simulink model "Microgrid_PV_WG_Bat_EV_j_22b"  (R2022b)
settings: Solver=VariableStepAuto  StartTime=0.0  StopTime=1  RelTol=1e-3
undefined symbols (not defined in the file or in its folder): Acid, Ion, Lead, Lithium
libraries: slpidlib x35, spsabctodq0Lib x23, spsSeriesRLCBranchLib x19, spsCurrentMeasurementLib x13, spsVoltageMeasurementLib x11, spsThreePhaseVIMeasurementLib x10, spsPLL3phLib x9, spsThreePhaseSeriesRLCBranchLib x9, spsPower3phInstantaneousLib x8, spsIGBTDiodeLib x8, spsUniversalBridgeLib x7, spsPWMGeneratorDCDCLib x6
(part 4 of 5)

== system Microgrid_PV_WG_Bat_EV_j_22b/逆变器整流1/controller2 ==
  note: abc2dq
  Udc : Inport
  Udc_ref : Inport  Port=2
  Vabc : Inport  Port=3
  Iabc : Inport  Port=4
  Constant : Constant  Commented=on  Value=600
  Constant4 : Constant  Value=0
  Demux2 : Demux  Outputs=3
  Demux3 : Demux  Outputs=3
  Demux4 : Demux  Outputs=3
  Gain6 : Gain  Gain=2*pi*50*(7e-3)
  Gain7 : Gain  Gain=2*pi*50*(7e-3)
  Gain9 : Gain  Gain=0.0017
  Mux1 : Mux  Inputs=3
  PID 3 : slpidlib/PID Controller  Controller=PID  Form=Parallel  TimeDomain=Discrete-time  UseExternalTs=off  SampleTime=1e-5  IntegratorMethod=Forward Euler  FilterMethod=Forward Euler  ControllerParametersSource=internal  P=2  I=70  UseKiTs=off  D=0  N=100  UseFilter=on  TunerSelectOption=Transfer Function Based (PID Tuner App)  InitialConditionSource=internal  InitialConditionForIntegrator=0  InitialConditionForFilter=0  DifferentiatorICPrevScaledInput=0  ExternalReset=none  TrackingMode=off  Kt=1  LimitOutput=off  SatLimitsSource=internal  UpperSaturationLimit=inf  LowerSaturationLimit=-inf  LinearizeAsGain=on  AntiWindupMode=none  Kb=1  LimitIntegrator=off  UpperIntegratorSaturationLimit=inf  LowerIntegratorSaturationLimit=-inf  POutMin=[]  POutMax=[]  IOutMin=[]  IOutMax=[]  DOutMin=[]  DOutMax=[]  NOutMin=[]  NOutMax=[]  SumOutMin=[]  SumOutMax=[]  SaturationOutMin=[]  SaturationOutMax=[]  PParamMin=[]  PParamMax=[]  IParamMin=[]  IParamMax=[]  DParamMin=[]  DParamMax=[]  NParamMin=[]  NParamMax=[]  KbParamMin=[]  KbParamMax=[]  KtParamMin=[]  KtParamMax=[]  KbOutMin=[]  KbOutMax=[]  KtOutMin=[]  KtOutMax=[]  IntegratorOutMin=[]  IntegratorOutMax=[]  FilterOutMin=[]  FilterOutMax=[]  SumI1OutMin=[]  SumI1OutMax=[]  SumI2OutMin=[]  SumI2OutMax=[]  SumI3OutMin=[]  SumI3OutMax=[]  SumI4OutMin=[]  SumI4OutMax=[]  SumDOutMin=[]  SumDOutMax=[]  DifferentiatorOutMin=[]  DifferentiatorOutMax=[]  FilterDiffOutCoefMin=[]  FilterDiffOutCoefMax=[]  ReciprocalOutMin=[]  ReciprocalOutMax=[]  SumDenOutMin=[]  SumDenOutMax=[]  SumNumOutMin=[]  SumNumOutMax=[]  DivideOutMin=[]  DivideOutMax=[]  UdiffTsProdOutMin=[]  UdiffTsProdOutMax=[]  NTsProdOutMin=[]  NTsProdOutMax=[]  UintegralTsProdOutMin=[]  UintegralTsProdOutMax=[]  UngainTsProdOutMin=[]  UngainTsProdOutMax=[]  IntegratorContinuousStateAttributes=''  IntegratorStateMustResolveToSignalObject=off  IntegratorRTWStateStorageClass=Auto  FilterContinuousStateAttributes=''  FilterStateMustResolveToSignalObject=off  FilterRTWStateStorageClass=Auto  ParallelPVariant=InternalParameters  IdealPVariant=Disabled  IVariant=InternalParameters  DVariant=InternalParameters  IntegratorVariant=Discrete  SatVariant=Disabled  AWVariant=Passthrough  PCopyVariant=Disabled  TRVariant=Disabled  FdbkBlocksVariant=Forward  IdealPFdbkVariant=Disabled  SatFdbkVariant=Disabled  DerivativeFilterVariant=ForwardEulerFilter  NVariant=InternalParameters  NCopyVariant=Disabled  FilterICVariant=InternalICsFilter  IntegratorICVariant=InternalICs  ExternalResetVariant=Disabled  TRSumVariant=Passthrough  SumFdbkVariant=Disabled  SumVariant=Sum_PID  TsampFilterVariant=InternalTs  TsampNgainVariant=Passthrough  TsampIntegralVariant=Disabled_SignalSpec  ExternalSaturationOutDataTypeStr=Inherit: Same as second input
  PID 4 : slpidlib/PID Controller  Controller=PID  Form=Parallel  TimeDomain=Discrete-time  UseExternalTs=off  SampleTime=1e-5  IntegratorMethod=Forward Euler  FilterMethod=Forward Euler  ControllerParametersSource=internal  P=10  I=0  UseKiTs=off  D=0  N=100  UseFilter=on  TunerSelectOption=Transfer Function Based (PID Tuner App)  InitialConditionSource=internal  InitialConditionForIntegrator=0  InitialConditionForFilter=0  DifferentiatorICPrevScaledInput=0  ExternalReset=none  TrackingMode=off  Kt=1  LimitOutput=off  SatLimitsSource=internal  UpperSaturationLimit=inf  LowerSaturationLimit=-inf  LinearizeAsGain=on  AntiWindupMode=none  Kb=1  LimitIntegrator=off  UpperIntegratorSaturationLimit=inf  LowerIntegratorSaturationLimit=-inf  POutMin=[]  POutMax=[]  IOutMin=[]  IOutMax=[]  DOutMin=[]  DOutMax=[]  NOutMin=[]  NOutMax=[]  SumOutMin=[]  SumOutMax=[]  SaturationOutMin=[]  SaturationOutMax=[]  PParamMin=[]  PParamMax=[]  IParamMin=[]  IParamMax=[]  DParamMin=[]  DParamMax=[]  NParamMin=[]  NParamMax=[]  KbParamMin=[]  KbParamMax=[]  KtParamMin=[]  KtParamMax=[]  KbOutMin=[]  KbOutMax=[]  KtOutMin=[]  KtOutMax=[]  IntegratorOutMin=[]  IntegratorOutMax=[]  FilterOutMin=[]  FilterOutMax=[]  SumI1OutMin=[]  SumI1OutMax=[]  SumI2OutMin=[]  SumI2OutMax=[]  SumI3OutMin=[]  SumI3OutMax=[]  SumI4OutMin=[]  SumI4OutMax=[]  SumDOutMin=[]  SumDOutMax=[]  DifferentiatorOutMin=[]  DifferentiatorOutMax=[]  FilterDiffOutCoefMin=[]  FilterDiffOutCoefMax=[]  ReciprocalOutMin=[]  ReciprocalOutMax=[]  SumDenOutMin=[]  SumDenOutMax=[]  SumNumOutMin=[]  SumNumOutMax=[]  DivideOutMin=[]  DivideOutMax=[]  UdiffTsProdOutMin=[]  UdiffTsProdOutMax=[]  NTsProdOutMin=[]  NTsProdOutMax=[]  UintegralTsProdOutMin=[]  UintegralTsProdOutMax=[]  UngainTsProdOutMin=[]  UngainTsProdOutMax=[]  IntegratorContinuousStateAttributes=''  IntegratorStateMustResolveToSignalObject=off  IntegratorRTWStateStorageClass=Auto  FilterContinuousStateAttributes=''  FilterStateMustResolveToSignalObject=off  FilterRTWStateStorageClass=Auto  ParallelPVariant=InternalParameters  IdealPVariant=Disabled  IVariant=InternalParameters  DVariant=InternalParameters  IntegratorVariant=Discrete  SatVariant=Disabled  AWVariant=Passthrough  PCopyVariant=Disabled  TRVariant=Disabled  FdbkBlocksVariant=Forward  IdealPFdbkVariant=Disabled  SatFdbkVariant=Disabled  DerivativeFilterVariant=ForwardEulerFilter  NVariant=InternalParameters  NCopyVariant=Disabled  FilterICVariant=InternalICsFilter  IntegratorICVariant=InternalICs  ExternalResetVariant=Disabled  TRSumVariant=Passthrough  SumFdbkVariant=Disabled  SumVariant=Sum_PID  TsampFilterVariant=InternalTs  TsampNgainVariant=Passthrough  TsampIntegralVariant=Disabled_SignalSpec  ExternalSaturationOutDataTypeStr=Inherit: Same as second input
  PID 5 : slpidlib/PID Controller  Controller=PID  Form=Parallel  TimeDomain=Discrete-time  UseExternalTs=off  SampleTime=1e-5  IntegratorMethod=Forward Euler  FilterMethod=Forward Euler  ControllerParametersSource=internal  P=10  I=0  UseKiTs=off  D=0  N=100  UseFilter=on  TunerSelectOption=Transfer Function Based (PID Tuner App)  InitialConditionSource=internal  InitialConditionForIntegrator=0  InitialConditionForFilter=0  DifferentiatorICPrevScaledInput=0  ExternalReset=none  TrackingMode=off  Kt=1  LimitOutput=off  SatLimitsSource=internal  UpperSaturationLimit=inf  LowerSaturationLimit=-inf  LinearizeAsGain=on  AntiWindupMode=none  Kb=1  LimitIntegrator=off  UpperIntegratorSaturationLimit=inf  LowerIntegratorSaturationLimit=-inf  POutMin=[]  POutMax=[]  IOutMin=[]  IOutMax=[]  DOutMin=[]  DOutMax=[]  NOutMin=[]  NOutMax=[]  SumOutMin=[]  SumOutMax=[]  SaturationOutMin=[]  SaturationOutMax=[]  PParamMin=[]  PParamMax=[]  IParamMin=[]  IParamMax=[]  DParamMin=[]  DParamMax=[]  NParamMin=[]  NParamMax=[]  KbParamMin=[]  KbParamMax=[]  KtParamMin=[]  KtParamMax=[]  KbOutMin=[]  KbOutMax=[]  KtOutMin=[]  KtOutMax=[]  IntegratorOutMin=[]  IntegratorOutMax=[]  FilterOutMin=[]  FilterOutMax=[]  SumI1OutMin=[]  SumI1OutMax=[]  SumI2OutMin=[]  SumI2OutMax=[]  SumI3OutMin=[]  SumI3OutMax=[]  SumI4OutMin=[]  SumI4OutMax=[]  SumDOutMin=[]  SumDOutMax=[]  DifferentiatorOutMin=[]  DifferentiatorOutMax=[]  FilterDiffOutCoefMin=[]  FilterDiffOutCoefMax=[]  ReciprocalOutMin=[]  ReciprocalOutMax=[]  SumDenOutMin=[]  SumDenOutMax=[]  SumNumOutMin=[]  SumNumOutMax=[]  DivideOutMin=[]  DivideOutMax=[]  UdiffTsProdOutMin=[]  UdiffTsProdOutMax=[]  NTsProdOutMin=[]  NTsProdOutMax=[]  UintegralTsProdOutMin=[]  UintegralTsProdOutMax=[]  UngainTsProdOutMin=[]  UngainTsProdOutMax=[]  IntegratorContinuousStateAttributes=''  IntegratorStateMustResolveToSignalObject=off  IntegratorRTWStateStorageClass=Auto  FilterContinuousStateAttributes=''  FilterStateMustResolveToSignalObject=off  FilterRTWStateStorageClass=Auto  ParallelPVariant=InternalParameters  IdealPVariant=Disabled  IVariant=InternalParameters  DVariant=InternalParameters  IntegratorVariant=Discrete  SatVariant=Disabled  AWVariant=Passthrough  PCopyVariant=Disabled  TRVariant=Disabled  FdbkBlocksVariant=Forward  IdealPFdbkVariant=Disabled  SatFdbkVariant=Disabled  DerivativeFilterVariant=ForwardEulerFilter  NVariant=InternalParameters  NCopyVariant=Disabled  FilterICVariant=InternalICsFilter  IntegratorICVariant=InternalICs  ExternalResetVariant=Disabled  TRSumVariant=Passthrough  SumFdbkVariant=Disabled  SumVariant=Sum_PID  TsampFilterVariant=InternalTs  TsampNgainVariant=Passthrough  TsampIntegralVariant=Disabled_SignalSpec  ExternalSaturationOutDataTypeStr=Inherit: Same as second input
  PLL (3ph)1 : spsPLL3phLib/PLL (3ph)  Fmin=45  Par_Init=[0, 50]  ParK=[180, 3200, 1]  TcD=1e-4  MaxRateChangeFreq=12  FilterCutOffFreq=25  Ts=0  AGC=on
  SVPWM Generator (2-Level)1 : spsSVPWMGenerator2LevelLib/SVPWM Generator (2-Level)  InputType=alpha-beta components  SwitchingPattern=Pattern #1  Fc=10000  ParUref=[0.8 -30 50]  Ts=0
  Scope : Scope  NumInputPorts=2
  Scope1 : Scope  NumInputPorts=2
  Sum1 : Sum  Commented=on  Inputs=|+-
  Sum5 : Sum  Inputs=|+-
  Sum6 : Sum  Inputs=|+-
  Sum7 : Sum  Inputs=++-
  Sum8 : Sum  Inputs=-+|
  Sum9 : Sum  Inputs=+++
  Terminator2 : Terminator
  Terminator3 : Terminator
  Terminator4 : Terminator
  abc to dq1 : spsabctodq0Lib/abc to dq0  Alignment=90 degrees behind phase A axis
  abc to dq2 : spsabctodq0Lib/abc to dq0  Alignment=90 degrees behind phase A axis
  dq0 to Alpha-Beta-Zero1 : spsdq0toAlphaBetaZeroLib/dq0 to Alpha-Beta-Zero  Alignment=90 degrees behind phase A axis
  iq*=0 : Constant  Value=0
  Pulse : Outport
  wires:
  Sum5/1 -> PID 3/1
  Gain6/1 -> Sum7/3
  Demux2/1 -> Sum7/1  "Vd"
  PID 3/1 -> Scope1/1, Sum6/1  "id*"
  dq0 to Alpha-Beta-Zero1/1 -> Gain9/1
  PLL (3ph)1/2 -> dq0 to Alpha-Beta-Zero1/2, abc to dq2/2, abc to dq1/2
  Sum6/1 -> PID 4/1
  PID 4/1 -> Sum7/2
  Demux4/3 -> Terminator4/1
  PID 5/1 -> Sum9/2
  Iabc/1 -> abc to dq2/1
  Constant4/1 -> Mux1/3
  Demux3/3 -> Terminator3/1
  abc to dq1/1 -> Demux2/1
  Demux2/3 -> Terminator2/1
  Udc/1 -> Sum5/1
  abc to dq2/1 -> Demux3/1
  iq*=0/1 -> Scope/2, Sum8/2
  SVPWM Generator (2-Level)1/1 -> Pulse/1
  Gain9/1 -> Demux4/1
  Demux3/2 -> Scope/1, Sum8/1, Gain6/1  "iq"
  Demux3/1 -> Gain7/1, Scope1/2, Sum6/2  "id"
  Sum7/1 -> Mux1/1  "Ud*"
  Sum8/1 -> PID 5/1
  Sum9/1 -> Mux1/2  "Uq*"
  Mux1/1 -> dq0 to Alpha-Beta-Zero1/1
  Demux4/1 -> SVPWM Generator (2-Level)1/1
  Demux4/2 -> SVPWM Generator (2-Level)1/2
  Udc_ref/1 -> Sum5/2
  Gain7/1 -> Sum9/3
  Demux2/2 -> Sum9/1  "Vq"
  Vabc/1 -> PLL (3ph)1/1, abc to dq1/1  "d"
  Constant/1 -> Sum1/2

== system Microgrid_PV_WG_Bat_EV_j_22b/DC//AC2/PQ/PQ控制 ==
  Vd : Inport
  Vq : Inport  Port=2
  P : Inport  Port=3
  Q : Inport  Port=4
  Add : Sum
  Add1 : Sum
  Add2 : Sum  Inputs=+-
  Divide : Product  Inputs=*/
  Divide1 : Product  Inputs=/*
  Gain2 : Gain  Gain=2/3
  Gain3 : Gain  Gain=2/3
  Product{1..2,7..10} (6 alike) : Product
  Id_ref : Outport
  Iq_ref : Outport  Port=2
  wires:
  Gain2/1 -> Divide/1
  Q/1 -> Product10/2, Product2/2
  Vq/1 -> Product9/1, Product8/2, Product8/1, Product2/1
  Product8/1 -> Add1/2
  Add/1 -> Gain2/1
  Product1/1 -> Add/1
  Product10/1 -> Add2/2
  Gain3/1 -> Divide1/2
  Divide/1 -> Id_ref/1  "Id_ref"
  P/1 -> Product9/2, Product1/2
  Product9/1 -> Add2/1
  Vd/1 -> Product7/2, Product7/1, Product10/1, Product1/1
  Divide1/1 -> Iq_ref/1  "Iq_ref"
  Product2/1 -> Add/2
  Add1/1 -> Divide1/1, Divide/2
  Add2/1 -> Gain3/1
  Product7/1 -> Add1/1

== system Microgrid_PV_WG_Bat_EV_j_22b/DC//AC2/PQ/功率控制1 ==
  Vd : Inport
  Vq : Inport  Port=2
  Id : Inport  Port=3
  Iq : Inport  Port=4
  Add : Sum
  Add1 : Sum
  Product{1..2,7..8} (4 alike) : Product
  Transfer Fcn : TransferFcn  Numerator=[40]  Denominator=[1 40]
  Transfer Fcn1 : TransferFcn  Numerator=[40]  Denominator=[1 40]
  P : Outport
  Q : Outport  Port=2
  wires:
  Product2/1 -> Add/2
  Product1/1 -> Add/1
  Add/1 -> Transfer Fcn1/1
  Product8/1 -> Add1/2
  Product7/1 -> Add1/1
  Vd/1 -> Product2/1, Product7/1
  Id/1 -> Product7/2, Product1/2
  Iq/1 -> Product8/2, Product2/2
  Vq/1 -> Product1/1, Product8/1
  Add1/1 -> Transfer Fcn/1
  Transfer Fcn/1 -> P/1
  Transfer Fcn1/1 -> Q/1

== system Microgrid_PV_WG_Bat_EV_j_22b/DC//AC2/PQ/坐标变换1 ==
  ILabc : Inport
  Vabc : Inport  Port=2
  Iabc : Inport  Port=3
  wt : Inport  Port=4
  Demux : Demux  Outputs=3
  Demux1 : Demux  Outputs=3
  Demux2 : Demux  Outputs=3
  Terminator : Terminator
  Terminator1 : Terminator
  Terminator2 : Terminator
  abc to dq0 : spsabctodq0Lib/abc to dq0  Alignment=90 degrees behind phase A axis
  abc to dq1 : spsabctodq0Lib/abc to dq0  Alignment=90 degrees behind phase A axis
  abc to dq2 : spsabctodq0Lib/abc to dq0  Alignment=90 degrees behind phase A axis
  ILd : Outport
  ILq : Outport  Port=2
  Vd : Outport  Port=3
  Vq : Outport  Port=4
  Id : Outport  Port=5
  Iq : Outport  Port=6
  wires:
  ILabc/1 -> abc to dq0/1
  abc to dq0/1 -> Demux/1
  Demux/3 -> Terminator/1
  Demux/1 -> ILd/1
  Demux/2 -> ILq/1
  Demux1/2 -> Vq/1
  Demux1/1 -> Vd/1
  Demux1/3 -> Terminator1/1
  abc to dq1/1 -> Demux1/1
  Vabc/1 -> abc to dq1/1
  Iabc/1 -> abc to dq2/1
  abc to dq2/1 -> Demux2/1
  Demux2/3 -> Terminator2/1
  Demux2/1 -> Id/1
  Demux2/2 -> Iq/1
  wt/1 -> abc to dq2/2, abc to dq1/2, abc to dq0/2

== system Microgrid_PV_WG_Bat_EV_j_22b/DC//AC2/PQ/电压电流双闭环1 ==
  Id_ref : Inport
  Iq_ref : Inport  Port=2
  Vd : Inport  Port=3
  Vq : Inport  Port=4
  Iq : Inport  Port=5
  Id : Inport  Port=6
  Vabc : Inport  Port=7
  Add6 : Sum  Inputs=|+-
  Add7 : Sum  Inputs=|+-
  Add8 : Sum  Inputs=+++
  Add9 : Sum  Inputs=++-
  Constant6 : Constant  Value=0
  Constant7 : Constant  Value=3e-3
  Constant8 : Constant  Value=3e-3
  Gain : Gain  Gain=2*pi
  Gain1 : Gain  Gain=2*pi
  Mux1 : Mux  Inputs=3
  PID Controller1 : slpidlib/PID Controller  Controller=PI  Form=Parallel  TimeDomain=Discrete-time  UseExternalTs=off  SampleTime=1e-5  IntegratorMethod=Forward Euler  FilterMethod=Forward Euler  ControllerParametersSource=internal  P=200  I=500  UseKiTs=off  D=0  N=100  UseFilter=on  TunerSelectOption=Transfer Function Based (PID Tuner App)  InitialConditionSource=internal  InitialConditionForIntegrator=0  InitialConditionForFilter=0  DifferentiatorICPrevScaledInput=0  ExternalReset=none  TrackingMode=off  Kt=1  LimitOutput=off  SatLimitsSource=internal  UpperSaturationLimit=inf  LowerSaturationLimit=-inf  LinearizeAsGain=on  AntiWindupMode=none  Kb=1  LimitIntegrator=off  UpperIntegratorSaturationLimit=inf  LowerIntegratorSaturationLimit=-inf  POutMin=[]  POutMax=[]  IOutMin=[]  IOutMax=[]  DOutMin=[]  DOutMax=[]  NOutMin=[]  NOutMax=[]  SumOutMin=[]  SumOutMax=[]  SaturationOutMin=[]  SaturationOutMax=[]  PParamMin=[]  PParamMax=[]  IParamMin=[]  IParamMax=[]  DParamMin=[]  DParamMax=[]  NParamMin=[]  NParamMax=[]  KbParamMin=[]  KbParamMax=[]  KtParamMin=[]  KtParamMax=[]  KbOutMin=[]  KbOutMax=[]  KtOutMin=[]  KtOutMax=[]  IntegratorOutMin=[]  IntegratorOutMax=[]  FilterOutMin=[]  FilterOutMax=[]  SumI1OutMin=[]  SumI1OutMax=[]  SumI2OutMin=[]  SumI2OutMax=[]  SumI3OutMin=[]  SumI3OutMax=[]  SumI4OutMin=[]  SumI4OutMax=[]  SumDOutMin=[]  SumDOutMax=[]  DifferentiatorOutMin=[]  DifferentiatorOutMax=[]  FilterDiffOutCoefMin=[]  FilterDiffOutCoefMax=[]  ReciprocalOutMin=[]  ReciprocalOutMax=[]  SumDenOutMin=[]  SumDenOutMax=[]  SumNumOutMin=[]  SumNumOutMax=[]  DivideOutMin=[]  DivideOutMax=[]  UdiffTsProdOutMin=[]  UdiffTsProdOutMax=[]  NTsProdOutMin=[]  NTsProdOutMax=[]  UintegralTsProdOutMin=[]  UintegralTsProdOutMax=[]  UngainTsProdOutMin=[]  UngainTsProdOutMax=[]  IntegratorContinuousStateAttributes=''  IntegratorStateMustResolveToSignalObject=off  IntegratorRTWStateStorageClass=Auto  FilterContinuousStateAttributes=''  FilterStateMustResolveToSignalObject=off  FilterRTWStateStorageClass=Auto  ParallelPVariant=InternalParameters  IdealPVariant=Disabled  IVariant=InternalParameters  DVariant=Disabled  IntegratorVariant=Discrete  SatVariant=Disabled  AWVariant=Passthrough  PCopyVariant=Disabled  TRVariant=Disabled  FdbkBlocksVariant=Forward  IdealPFdbkVariant=Disabled  SatFdbkVariant=Disabled  DerivativeFilterVariant=Disabled  NVariant=Disabled  NCopyVariant=Disabled_SignalSpec  FilterICVariant=Disabled  IntegratorICVariant=InternalICs  ExternalResetVariant=Disabled  TRSumVariant=Passthrough  SumFdbkVariant=Disabled  SumVariant=Sum_PI  TsampFilterVariant=InternalTs  TsampNgainVariant=Passthrough  TsampIntegralVariant=Disabled_SignalSpec  ExternalSaturationOutDataTypeStr=Inherit: Same as second input
  PID Controller2 : slpidlib/PID Controller  Controller=PI  Form=Parallel  TimeDomain=Discrete-time  UseExternalTs=off  SampleTime=1e-5  IntegratorMethod=Forward Euler  FilterMethod=Forward Euler  ControllerParametersSource=internal  P=200  I=500  UseKiTs=off  D=0  N=100  UseFilter=on  TunerSelectOption=Transfer Function Based (PID Tuner App)  InitialConditionSource=internal  InitialConditionForIntegrator=0  InitialConditionForFilter=0  DifferentiatorICPrevScaledInput=0  ExternalReset=none  TrackingMode=off  Kt=1  LimitOutput=off  SatLimitsSource=internal  UpperSaturationLimit=inf  LowerSaturationLimit=-inf  LinearizeAsGain=on  AntiWindupMode=none  Kb=1  LimitIntegrator=off  UpperIntegratorSaturationLimit=inf  LowerIntegratorSaturationLimit=-inf  POutMin=[]  POutMax=[]  IOutMin=[]  IOutMax=[]  DOutMin=[]  DOutMax=[]  NOutMin=[]  NOutMax=[]  SumOutMin=[]  SumOutMax=[]  SaturationOutMin=[]  SaturationOutMax=[]  PParamMin=[]  PParamMax=[]  IParamMin=[]  IParamMax=[]  DParamMin=[]  DParamMax=[]  NParamMin=[]  NParamMax=[]  KbParamMin=[]  KbParamMax=[]  KtParamMin=[]  KtParamMax=[]  KbOutMin=[]  KbOutMax=[]  KtOutMin=[]  KtOutMax=[]  IntegratorOutMin=[]  IntegratorOutMax=[]  FilterOutMin=[]  FilterOutMax=[]  SumI1OutMin=[]  SumI1OutMax=[]  SumI2OutMin=[]  SumI2OutMax=[]  SumI3OutMin=[]  SumI3OutMax=[]  SumI4OutMin=[]  SumI4OutMax=[]  SumDOutMin=[]  SumDOutMax=[]  DifferentiatorOutMin=[]  DifferentiatorOutMax=[]  FilterDiffOutCoefMin=[]  FilterDiffOutCoefMax=[]  ReciprocalOutMin=[]  ReciprocalOutMax=[]  SumDenOutMin=[]  SumDenOutMax=[]  SumNumOutMin=[]  SumNumOutMax=[]  DivideOutMin=[]  DivideOutMax=[]  UdiffTsProdOutMin=[]  UdiffTsProdOutMax=[]  NTsProdOutMin=[]  NTsProdOutMax=[]  UintegralTsProdOutMin=[]  UintegralTsProdOutMax=[]  UngainTsProdOutMin=[]  UngainTsProdOutMax=[]  IntegratorContinuousStateAttributes=''  IntegratorStateMustResolveToSignalObject=off  IntegratorRTWStateStorageClass=Auto  FilterContinuousStateAttributes=''  FilterStateMustResolveToSignalObject=off  FilterRTWStateStorageClass=Auto  ParallelPVariant=InternalParameters  IdealPVariant=Disabled  IVariant=InternalParameters  DVariant=Disabled  IntegratorVariant=Discrete  SatVariant=Disabled  AWVariant=Passthrough  PCopyVariant=Disabled  TRVariant=Disabled  FdbkBlocksVariant=Forward  IdealPFdbkVariant=Disabled  SatFdbkVariant=Disabled  DerivativeFilterVariant=Disabled  NVariant=Disabled  NCopyVariant=Disabled_SignalSpec  FilterICVariant=Disabled  IntegratorICVariant=InternalICs  ExternalResetVariant=Disabled  TRSumVariant=Passthrough  SumFdbkVariant=Disabled  SumVariant=Sum_PI  TsampFilterVariant=InternalTs  TsampNgainVariant=Passthrough  TsampIntegralVariant=Disabled_SignalSpec  ExternalSaturationOutDataTypeStr=Inherit: Same as second input
  PLL (3ph)1 : spsPLL3phLib/PLL (3ph)  Fmin=45  Par_Init=[0, 50]  ParK=[180, 3200, 1]  TcD=1e-4  MaxRateChangeFreq=12  FilterCutOffFreq=25  Ts=0  AGC=on
  PWM Generator (2-Level)1 : spsPWMGenerator2LevelLib/PWM Generator (2-Level)  ModulatorType=Three-phase bridge (6 pulses)  ModulatorMode=Unsynchronized  Fc=100*50  Pc=90  nF=27  MinMax="[ -1  1 ]"  SamplingTechnique=Natural  ModulatingSignals=off  m=0.8  Freq=60  Phase=0  Ts=0  ShowCarrierOutport=off
  Product{3..6} (4 alike) : Product
  dq0 to abc1 : spsdq0toabcLib/dq0 to abc  Alignment=90 degrees behind phase A axis
  PWM : Outport
  wt : Outport  Port=2
  wires:
  Vd/1 -> Add8/3
  Iq_ref/1 -> Add7/1
  Id_ref/1 -> Add6/1
  Add7/1 -> PID Controller2/1
  Constant6/1 -> Mux1/3
  PID Controller2/1 -> Add9/2
  Product6/1 -> Add9/3
  Add8/1 -> Mux1/1
  Vq/1 -> Add9/1
  dq0 to abc1/1 -> PWM Generator (2-Level)1/1
  Product4/1 -> Add8/1
  Add6/1 -> PID Controller1/1
  Add9/1 -> Mux1/2
  PID Controller1/1 -> Add8/2
  Id/1 -> Add6/2, Product6/1
  PWM Generator (2-Level)1/1 -> PWM/1
  Constant7/1 -> Product3/2
  Iq/1 -> Product4/2, Add7/2
  Mux1/1 -> dq0 to abc1/1
  Product3/1 -> Product4/1
  Constant8/1 -> Product5/2
  Product5/1 -> Product6/2
  [wt] -> dq0 to abc1/2
  [f] -> Gain1/1, Gain/1
  Gain/1 -> Product3/1
  Gain1/1 -> Product5/1
  PLL (3ph)1/1 -> [f]
  Vabc/1 -> PLL (3ph)1/1
  PLL (3ph)1/2 -> wt/1, [wt]

== system Microgrid_PV_WG_Bat_EV_j_22b/DC//AC2/V//F/V//F控制 ==
  Vset : Inport
  f_set : Inport  Port=2
  Add : Sum
  Constant1 : Constant  Value=2*pi
  Constant5 : Constant  Value=[0 -2*pi/3 2*pi/3]
  Demux1 : Demux  Outputs=3
  Integrator1 : Integrator
  Mod2 : Math  Operator=mod
  Product1 : Product
  Scope3 : Scope
  Sin1 : Trigonometry
  Sum2 : Sum  Inputs=|++
  Terminator1 : Terminator
  abc to dq1 : spsabctodq0Lib/abc to dq0  Alignment=90 degrees behind phase A axis
  gain : Gain  Gain=2*pi
  Vd_ref : Outport
  Vq_ref : Outport  Port=2
  wt : Outport  Port=3
  wires:
  [delta_theta_comp] -> Add/1
  Add/1 -> wt/1, Scope3/1, abc to dq1/2, Sum2/1
  Product1/1 -> abc to dq1/1
  f_set/1 -> gain/1
  Sin1/1 -> Product1/1
  Vset/1 -> Product1/2
  Integrator1/1 -> Mod2/1
  Demux1/3 -> Terminator1/1
  Mod2/1 -> Add/2  "wt"
  Constant5/1 -> Sum2/2
  Constant1/1 -> Mod2/2
  gain/1 -> Integrator1/1
  Demux1/1 -> Vd_ref/1
  abc to dq1/1 -> Demux1/1
  Demux1/2 -> Vq_ref/1
  Sum2/1 -> Sin1/1

== system Microgrid_PV_WG_Bat_EV_j_22b/DC//AC2/V//F/功率控制 ==
  Vd : Inport
  Vq : Inport  Port=2
  Id : Inport  Port=3
  Iq : Inport  Port=4
  Add : Sum
  Add1 : Sum
  Product{1..2,7..8} (4 alike) : Product
  Transfer Fcn : TransferFcn  Numerator=[40]  Denominator=[1 40]
  Transfer Fcn1 : TransferFcn  Numerator=[40]  Denominator=[1 40]
  P : Outport
  Q : Outport  Port=2
  wires:
  Product2/1 -> Add/2
  Product1/1 -> Add/1
  Add/1 -> Transfer Fcn1/1
  Product8/1 -> Add1/2
  Product7/1 -> Add1/1
  Vd/1 -> Product2/1, Product7/1
  Id/1 -> Product7/2, Product1/2
  Iq/1 -> Product8/2, Product2/2
  Vq/1 -> Product1/1, Product8/1
  Add1/1 -> Transfer Fcn/1
  Transfer Fcn/1 -> P/1
  Transfer Fcn1/1 -> Q/1

== system Microgrid_PV_WG_Bat_EV_j_22b/DC//AC2/V//F/坐标变换 ==
  ILabc : Inport
  Vabc : Inport  Port=2
  Iabc : Inport  Port=3
  wt : Inport  Port=4
  Demux : Demux  Outputs=3
  Demux1 : Demux  Outputs=3
  Demux2 : Demux  Outputs=3
  Terminator : Terminator
  Terminator1 : Terminator
  Terminator2 : Terminator
  abc to dq0 : spsabctodq0Lib/abc to dq0  Alignment=90 degrees behind phase A axis
  abc to dq1 : spsabctodq0Lib/abc to dq0  Alignment=90 degrees behind phase A axis
  abc to dq2 : spsabctodq0Lib/abc to dq0  Alignment=90 degrees behind phase A axis
  ILd : Outport
  ILq : Outport  Port=2
  Vd : Outport  Port=3
  Vq : Outport  Port=4
  Id : Outport  Port=5
  Iq : Outport  Port=6
  wires:
  ILabc/1 -> abc to dq0/1
  abc to dq0/1 -> Demux/1
  Demux/3 -> Terminator/1
  Demux/1 -> ILd/1
  Demux/2 -> ILq/1
  Demux1/2 -> Vq/1
  Demux1/1 -> Vd/1
  Demux1/3 -> Terminator1/1
  abc to dq1/1 -> Demux1/1
  Vabc/1 -> abc to dq1/1
  Iabc/1 -> abc to dq2/1
  abc to dq2/1 -> Demux2/1
  Demux2/3 -> Terminator2/1
  Demux2/1 -> Id/1
  Demux2/2 -> Iq/1
  wt/1 -> abc to dq2/2, abc to dq1/2, abc to dq0/2

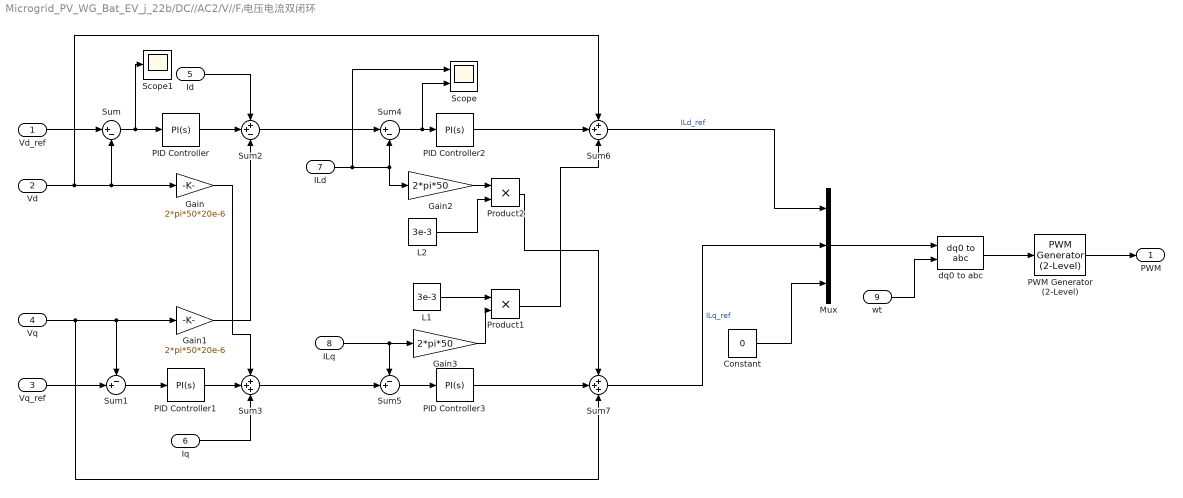
== system Microgrid_PV_WG_Bat_EV_j_22b/DC//AC2/V//F/电压电流双闭环 ==
  Vd_ref : Inport
  Vd : Inport  Port=2
  Vq_ref : Inport  Port=3
  Vq : Inport  Port=4
  Id : Inport  Port=5
  Iq : Inport  Port=6
  ILd : Inport  Port=7
  ILq : Inport  Port=8
  wt : Inport  Port=9
  Constant : Constant  Value=0
  Gain : Gain  Gain=2*pi*50*20e-6
  Gain1 : Gain  Gain=2*pi*50*20e-6
  Gain2 : Gain  Gain=2*pi*50
  Gain3 : Gain  Gain=2*pi*50
  L1 : Constant  Value=3e-3
  L2 : Constant  Value=3e-3
  Mux : Mux  Inputs=3
  PID Controller : slpidlib/PID Controller  Controller=PI  Form=Parallel  TimeDomain=Continuous-time  UseExternalTs=off  SampleTime=-1  IntegratorMethod=Forward Euler  FilterMethod=Forward Euler  ControllerParametersSource=internal  P=0.4  I=10  UseKiTs=off  D=0  N=100  UseFilter=on  TunerSelectOption=Transfer Function Based (PID Tuner App)  InitialConditionSource=internal  InitialConditionForIntegrator=0  InitialConditionForFilter=0  DifferentiatorICPrevScaledInput=0  ExternalReset=none  TrackingMode=off  Kt=1  LimitOutput=off  SatLimitsSource=internal  UpperSaturationLimit=inf  LowerSaturationLimit=-inf  LinearizeAsGain=on  AntiWindupMode=none  Kb=1  LimitIntegrator=off  UpperIntegratorSaturationLimit=inf  LowerIntegratorSaturationLimit=-inf  POutMin=[]  POutMax=[]  IOutMin=[]  IOutMax=[]  DOutMin=[]  DOutMax=[]  NOutMin=[]  NOutMax=[]  SumOutMin=[]  SumOutMax=[]  SaturationOutMin=[]  SaturationOutMax=[]  PParamMin=[]  PParamMax=[]  IParamMin=[]  IParamMax=[]  DParamMin=[]  DParamMax=[]  NParamMin=[]  NParamMax=[]  KbParamMin=[]  KbParamMax=[]  KtParamMin=[]  KtParamMax=[]  KbOutMin=[]  KbOutMax=[]  KtOutMin=[]  KtOutMax=[]  IntegratorOutMin=[]  IntegratorOutMax=[]  FilterOutMin=[]  FilterOutMax=[]  SumI1OutMin=[]  SumI1OutMax=[]  SumI2OutMin=[]  SumI2OutMax=[]  SumI3OutMin=[]  SumI3OutMax=[]  SumI4OutMin=[]  SumI4OutMax=[]  SumDOutMin=[]  SumDOutMax=[]  DifferentiatorOutMin=[]  DifferentiatorOutMax=[]  FilterDiffOutCoefMin=[]  FilterDiffOutCoefMax=[]  ReciprocalOutMin=[]  ReciprocalOutMax=[]  SumDenOutMin=[]  SumDenOutMax=[]  SumNumOutMin=[]  SumNumOutMax=[]  DivideOutMin=[]  DivideOutMax=[]  UdiffTsProdOutMin=[]  UdiffTsProdOutMax=[]  NTsProdOutMin=[]  NTsProdOutMax=[]  UintegralTsProdOutMin=[]  UintegralTsProdOutMax=[]  UngainTsProdOutMin=[]  UngainTsProdOutMax=[]  IntegratorContinuousStateAttributes=''  IntegratorStateMustResolveToSignalObject=off  IntegratorRTWStateStorageClass=Auto  FilterContinuousStateAttributes=''  FilterStateMustResolveToSignalObject=off  FilterRTWStateStorageClass=Auto  ParallelPVariant=InternalParameters  IdealPVariant=Disabled  IVariant=InternalParameters  DVariant=Disabled  IntegratorVariant=Continuous  SatVariant=Disabled  AWVariant=Passthrough  PCopyVariant=Disabled  TRVariant=Disabled  FdbkBlocksVariant=Forward  IdealPFdbkVariant=Disabled  SatFdbkVariant=Disabled  DerivativeFilterVariant=Disabled  NVariant=Disabled  NCopyVariant=Disabled_SignalSpec  FilterICVariant=Disabled  IntegratorICVariant=InternalICs  ExternalResetVariant=Disabled  TRSumVariant=Passthrough  SumFdbkVariant=Disabled  SumVariant=Sum_PI  TsampFilterVariant=InternalTs  TsampNgainVariant=Passthrough  TsampIntegralVariant=Disabled_SignalSpec  ExternalSaturationOutDataTypeStr=Inherit: Same as second input
  PID Controller1 : slpidlib/PID Controller  Controller=PI  Form=Parallel  TimeDomain=Continuous-time  UseExternalTs=off  SampleTime=-1  IntegratorMethod=Forward Euler  FilterMethod=Forward Euler  ControllerParametersSource=internal  P=0.4  I=10  UseKiTs=off  D=0  N=100  UseFilter=on  TunerSelectOption=Transfer Function Based (PID Tuner App)  InitialConditionSource=internal  InitialConditionForIntegrator=0  InitialConditionForFilter=0  DifferentiatorICPrevScaledInput=0  ExternalReset=none  TrackingMode=off  Kt=1  LimitOutput=off  SatLimitsSource=internal  UpperSaturationLimit=inf  LowerSaturationLimit=-inf  LinearizeAsGain=on  AntiWindupMode=none  Kb=1  LimitIntegrator=off  UpperIntegratorSaturationLimit=inf  LowerIntegratorSaturationLimit=-inf  POutMin=[]  POutMax=[]  IOutMin=[]  IOutMax=[]  DOutMin=[]  DOutMax=[]  NOutMin=[]  NOutMax=[]  SumOutMin=[]  SumOutMax=[]  SaturationOutMin=[]  SaturationOutMax=[]  PParamMin=[]  PParamMax=[]  IParamMin=[]  IParamMax=[]  DParamMin=[]  DParamMax=[]  NParamMin=[]  NParamMax=[]  KbParamMin=[]  KbParamMax=[]  KtParamMin=[]  KtParamMax=[]  KbOutMin=[]  KbOutMax=[]  KtOutMin=[]  KtOutMax=[]  IntegratorOutMin=[]  IntegratorOutMax=[]  FilterOutMin=[]  FilterOutMax=[]  SumI1OutMin=[]  SumI1OutMax=[]  SumI2OutMin=[]  SumI2OutMax=[]  SumI3OutMin=[]  SumI3OutMax=[]  SumI4OutMin=[]  SumI4OutMax=[]  SumDOutMin=[]  SumDOutMax=[]  DifferentiatorOutMin=[]  DifferentiatorOutMax=[]  FilterDiffOutCoefMin=[]  FilterDiffOutCoefMax=[]  ReciprocalOutMin=[]  ReciprocalOutMax=[]  SumDenOutMin=[]  SumDenOutMax=[]  SumNumOutMin=[]  SumNumOutMax=[]  DivideOutMin=[]  DivideOutMax=[]  UdiffTsProdOutMin=[]  UdiffTsProdOutMax=[]  NTsProdOutMin=[]  NTsProdOutMax=[]  UintegralTsProdOutMin=[]  UintegralTsProdOutMax=[]  UngainTsProdOutMin=[]  UngainTsProdOutMax=[]  IntegratorContinuousStateAttributes=''  IntegratorStateMustResolveToSignalObject=off  IntegratorRTWStateStorageClass=Auto  FilterContinuousStateAttributes=''  FilterStateMustResolveToSignalObject=off  FilterRTWStateStorageClass=Auto  ParallelPVariant=InternalParameters  IdealPVariant=Disabled  IVariant=InternalParameters  DVariant=Disabled  IntegratorVariant=Continuous  SatVariant=Disabled  AWVariant=Passthrough  PCopyVariant=Disabled  TRVariant=Disabled  FdbkBlocksVariant=Forward  IdealPFdbkVariant=Disabled  SatFdbkVariant=Disabled  DerivativeFilterVariant=Disabled  NVariant=Disabled  NCopyVariant=Disabled_SignalSpec  FilterICVariant=Disabled  IntegratorICVariant=InternalICs  ExternalResetVariant=Disabled  TRSumVariant=Passthrough  SumFdbkVariant=Disabled  SumVariant=Sum_PI  TsampFilterVariant=InternalTs  TsampNgainVariant=Passthrough  TsampIntegralVariant=Disabled_SignalSpec  ExternalSaturationOutDataTypeStr=Inherit: Same as second input
  PID Controller2 : slpidlib/PID Controller  Controller=PI  Form=Parallel  TimeDomain=Continuous-time  UseExternalTs=off  SampleTime=-1  IntegratorMethod=Forward Euler  FilterMethod=Forward Euler  ControllerParametersSource=internal  P=40  I=300  UseKiTs=off  D=0  N=100  UseFilter=on  TunerSelectOption=Transfer Function Based (PID Tuner App)  InitialConditionSource=internal  InitialConditionForIntegrator=0  InitialConditionForFilter=0  DifferentiatorICPrevScaledInput=0  ExternalReset=none  TrackingMode=off  Kt=1  LimitOutput=off  SatLimitsSource=internal  UpperSaturationLimit=inf  LowerSaturationLimit=-inf  LinearizeAsGain=on  AntiWindupMode=none  Kb=1  LimitIntegrator=off  UpperIntegratorSaturationLimit=inf  LowerIntegratorSaturationLimit=-inf  POutMin=[]  POutMax=[]  IOutMin=[]  IOutMax=[]  DOutMin=[]  DOutMax=[]  NOutMin=[]  NOutMax=[]  SumOutMin=[]  SumOutMax=[]  SaturationOutMin=[]  SaturationOutMax=[]  PParamMin=[]  PParamMax=[]  IParamMin=[]  IParamMax=[]  DParamMin=[]  DParamMax=[]  NParamMin=[]  NParamMax=[]  KbParamMin=[]  KbParamMax=[]  KtParamMin=[]  KtParamMax=[]  KbOutMin=[]  KbOutMax=[]  KtOutMin=[]  KtOutMax=[]  IntegratorOutMin=[]  IntegratorOutMax=[]  FilterOutMin=[]  FilterOutMax=[]  SumI1OutMin=[]  SumI1OutMax=[]  SumI2OutMin=[]  SumI2OutMax=[]  SumI3OutMin=[]  SumI3OutMax=[]  SumI4OutMin=[]  SumI4OutMax=[]  SumDOutMin=[]  SumDOutMax=[]  DifferentiatorOutMin=[]  DifferentiatorOutMax=[]  FilterDiffOutCoefMin=[]  FilterDiffOutCoefMax=[]  ReciprocalOutMin=[]  ReciprocalOutMax=[]  SumDenOutMin=[]  SumDenOutMax=[]  SumNumOutMin=[]  SumNumOutMax=[]  DivideOutMin=[]  DivideOutMax=[]  UdiffTsProdOutMin=[]  UdiffTsProdOutMax=[]  NTsProdOutMin=[]  NTsProdOutMax=[]  UintegralTsProdOutMin=[]  UintegralTsProdOutMax=[]  UngainTsProdOutMin=[]  UngainTsProdOutMax=[]  IntegratorContinuousStateAttributes=''  IntegratorStateMustResolveToSignalObject=off  IntegratorRTWStateStorageClass=Auto  FilterContinuousStateAttributes=''  FilterStateMustResolveToSignalObject=off  FilterRTWStateStorageClass=Auto  ParallelPVariant=InternalParameters  IdealPVariant=Disabled  IVariant=InternalParameters  DVariant=Disabled  IntegratorVariant=Continuous  SatVariant=Disabled  AWVariant=Passthrough  PCopyVariant=Disabled  TRVariant=Disabled  FdbkBlocksVariant=Forward  IdealPFdbkVariant=Disabled  SatFdbkVariant=Disabled  DerivativeFilterVariant=Disabled  NVariant=Disabled  NCopyVariant=Disabled_SignalSpec  FilterICVariant=Disabled  IntegratorICVariant=InternalICs  ExternalResetVariant=Disabled  TRSumVariant=Passthrough  SumFdbkVariant=Disabled  SumVariant=Sum_PI  TsampFilterVariant=InternalTs  TsampNgainVariant=Passthrough  TsampIntegralVariant=Disabled_SignalSpec  ExternalSaturationOutDataTypeStr=Inherit: Same as second input
  PID Controller3 : slpidlib/PID Controller  Controller=PI  Form=Parallel  TimeDomain=Continuous-time  UseExternalTs=off  SampleTime=-1  IntegratorMethod=Forward Euler  FilterMethod=Forward Euler  ControllerParametersSource=internal  P=40  I=300  UseKiTs=off  D=0  N=100  UseFilter=on  TunerSelectOption=Transfer Function Based (PID Tuner App)  InitialConditionSource=internal  InitialConditionForIntegrator=0  InitialConditionForFilter=0  DifferentiatorICPrevScaledInput=0  ExternalReset=none  TrackingMode=off  Kt=1  LimitOutput=off  SatLimitsSource=internal  UpperSaturationLimit=inf  LowerSaturationLimit=-inf  LinearizeAsGain=on  AntiWindupMode=none  Kb=1  LimitIntegrator=off  UpperIntegratorSaturationLimit=inf  LowerIntegratorSaturationLimit=-inf  POutMin=[]  POutMax=[]  IOutMin=[]  IOutMax=[]  DOutMin=[]  DOutMax=[]  NOutMin=[]  NOutMax=[]  SumOutMin=[]  SumOutMax=[]  SaturationOutMin=[]  SaturationOutMax=[]  PParamMin=[]  PParamMax=[]  IParamMin=[]  IParamMax=[]  DParamMin=[]  DParamMax=[]  NParamMin=[]  NParamMax=[]  KbParamMin=[]  KbParamMax=[]  KtParamMin=[]  KtParamMax=[]  KbOutMin=[]  KbOutMax=[]  KtOutMin=[]  KtOutMax=[]  IntegratorOutMin=[]  IntegratorOutMax=[]  FilterOutMin=[]  FilterOutMax=[]  SumI1OutMin=[]  SumI1OutMax=[]  SumI2OutMin=[]  SumI2OutMax=[]  SumI3OutMin=[]  SumI3OutMax=[]  SumI4OutMin=[]  SumI4OutMax=[]  SumDOutMin=[]  SumDOutMax=[]  DifferentiatorOutMin=[]  DifferentiatorOutMax=[]  FilterDiffOutCoefMin=[]  FilterDiffOutCoefMax=[]  ReciprocalOutMin=[]  ReciprocalOutMax=[]  SumDenOutMin=[]  SumDenOutMax=[]  SumNumOutMin=[]  SumNumOutMax=[]  DivideOutMin=[]  DivideOutMax=[]  UdiffTsProdOutMin=[]  UdiffTsProdOutMax=[]  NTsProdOutMin=[]  NTsProdOutMax=[]  UintegralTsProdOutMin=[]  UintegralTsProdOutMax=[]  UngainTsProdOutMin=[]  UngainTsProdOutMax=[]  IntegratorContinuousStateAttributes=''  IntegratorStateMustResolveToSignalObject=off  IntegratorRTWStateStorageClass=Auto  FilterContinuousStateAttributes=''  FilterStateMustResolveToSignalObject=off  FilterRTWStateStorageClass=Auto  ParallelPVariant=InternalParameters  IdealPVariant=Disabled  IVariant=InternalParameters  DVariant=Disabled  IntegratorVariant=Continuous  SatVariant=Disabled  AWVariant=Passthrough  PCopyVariant=Disabled  TRVariant=Disabled  FdbkBlocksVariant=Forward  IdealPFdbkVariant=Disabled  SatFdbkVariant=Disabled  DerivativeFilterVariant=Disabled  NVariant=Disabled  NCopyVariant=Disabled_SignalSpec  FilterICVariant=Disabled  IntegratorICVariant=InternalICs  ExternalResetVariant=Disabled  TRSumVariant=Passthrough  SumFdbkVariant=Disabled  SumVariant=Sum_PI  TsampFilterVariant=InternalTs  TsampNgainVariant=Passthrough  TsampIntegralVariant=Disabled_SignalSpec  ExternalSaturationOutDataTypeStr=Inherit: Same as second input
  PWM Generator (2-Level) : spsPWMGenerator2LevelLib/PWM Generator (2-Level)  ModulatorType=Three-phase bridge (6 pulses)  ModulatorMode=Unsynchronized  Fc=10e3  Pc=90  nF=27  MinMax="[ -1  1 ]"  SamplingTechnique=Natural  ModulatingSignals=off  m=0.8  Freq=60  Phase=0  Ts=0  ShowCarrierOutport=off
  Product1 : Product
  Product2 : Product
  Scope : Scope  NumInputPorts=2
  Scope1 : Scope
  Sum : Sum  Inputs=|+-
  Sum1 : Sum  Inputs=-+|
  Sum2 : Sum  Inputs=++-
  Sum3 : Sum  Inputs=+++
  Sum4 : Sum  Inputs=|+-
  Sum5 : Sum  Inputs=-+|
  Sum6 : Sum  Inputs=++-
  Sum7 : Sum  Inputs=+++
  dq0 to abc : spsdq0toabcLib/dq0 to abc  Alignment=90 degrees behind phase A axis
  PWM : Outport
  wires:
  Vd_ref/1 -> Sum/1
  Vd/1 -> Sum6/1, Sum/2, Gain/1
  Sum/1 -> Scope1/1, PID Controller/1
  Sum1/1 -> PID Controller1/1
  Vq/1 -> Sum7/3, Gain1/1, Sum1/1
  PID Controller/1 -> Sum2/2
  PID Controller1/1 -> Sum3/2
  Gain1/1 -> Sum2/3
  Id/1 -> Sum2/1
  ILd/1 -> Scope/1, Gain2/1, Sum4/2
  Sum4/1 -> Scope/2, PID Controller2/1
  Sum5/1 -> PID Controller3/1
  PID Controller2/1 -> Sum6/2
  PID Controller3/1 -> Sum7/2
  Gain2/1 -> Product2/1
  L2/1 -> Product2/2
  Gain/1 -> Sum3/1
  Iq/1 -> Sum3/3
  Vq_ref/1 -> Sum1/2
  Product2/1 -> Sum7/1
  L1/1 -> Product1/1
  Gain3/1 -> Product1/2
  ILq/1 -> Gain3/1, Sum5/1
  Product1/1 -> Sum6/3
  Sum6/1 -> Mux/1  "ILd_ref"
  Sum7/1 -> Mux/2  "ILq_ref"
  Constant/1 -> Mux/3
  Mux/1 -> dq0 to abc/1
  wt/1 -> dq0 to abc/2
  dq0 to abc/1 -> PWM Generator (2-Level)/1
  PWM Generator (2-Level)/1 -> PWM/1
  Sum2/1 -> Sum4/1
  Sum3/1 -> Sum5/2

== system Microgrid_PV_WG_Bat_EV_j_22b/DC//AC2/下垂控制/下垂控制 ==
  P : Inport
  Q : Inport  Port=2
  P_ref : Inport  Port=3
  Q_ref : Inport  Port=4
  Add : Sum
  Add1 : Sum
  Add2 : Sum
  Constant : Constant  Value=2*pi*50
  Constant1 : Constant  Value=2*pi
  Constant2 : Constant  Value=[0 -2*pi/3 2*pi/3]
  Constant3 : Constant  Value=600*sqrt(2)/sqrt(3)
  Demux : Demux  Outputs=3
  Integrator : Integrator
  KP : Gain  Gain=1.15e-4
  KQ : Gain  Gain=0.0025
  Mod : Math  Operator=mod
  Product : Product
  Sin : Trigonometry
  Sum : Sum  Inputs=|+-
  Sum1 : Sum  Inputs=|+-
  Terminator : Terminator
  abc to dq0 : spsabctodq0Lib/abc to dq0  Alignment=90 degrees behind phase A axis
  Vd_ref : Outport
  Vq_ref : Outport  Port=2
  wt : Outport  Port=3
  w : Outport  Port=4
  V : Outport  Port=5
  wires:
  P_ref/1 -> Sum/1
  P/1 -> Sum/2
  Q_ref/1 -> Sum1/1
  Q/1 -> Sum1/2
  Sum/1 -> KP/1
  Sum1/1 -> KQ/1
  KP/1 -> Add/1
  Constant/1 -> Add/2
  Add/1 -> w/1, Integrator/1  "w"
  Integrator/1 -> Mod/1
  Constant1/1 -> Mod/2
  Mod/1 -> wt/1, abc to dq0/2, Add1/1  "wt"
  Constant2/1 -> Add1/2
  Add1/1 -> Sin/1
  KQ/1 -> Add2/1
  Constant3/1 -> Add2/2
  Sin/1 -> Product/1
  Add2/1 -> V/1, Product/2
  Product/1 -> abc to dq0/1
  abc to dq0/1 -> Demux/1
  Demux/1 -> Vd_ref/1
  Demux/2 -> Vq_ref/1
  Demux/3 -> Terminator/1

== system Microgrid_PV_WG_Bat_EV_j_22b/DC//AC2/下垂控制/功率控制1 ==
  Vd : Inport
  Vq : Inport  Port=2
  Id : Inport  Port=3
  Iq : Inport  Port=4
  Add : Sum
  Add1 : Sum
  Product{1..2,7..8} (4 alike) : Product
  Transfer Fcn : TransferFcn  Numerator=[20]  Denominator=[1 20]
  Transfer Fcn1 : TransferFcn  Numerator=[20]  Denominator=[1 20]
  P : Outport
  Q : Outport  Port=2
  wires:
  Product2/1 -> Add/2
  Product1/1 -> Add/1
  Add/1 -> Transfer Fcn1/1
  Product8/1 -> Add1/2
  Product7/1 -> Add1/1
  Vd/1 -> Product2/1, Product7/1
  Id/1 -> Product7/2, Product1/2
  Iq/1 -> Product8/2, Product2/2
  Vq/1 -> Product1/1, Product8/1
  Add1/1 -> Transfer Fcn/1
  Transfer Fcn/1 -> P/1
  Transfer Fcn1/1 -> Q/1

== system Microgrid_PV_WG_Bat_EV_j_22b/DC//AC2/下垂控制/坐标变换1 ==
  ILabc : Inport
  Vabc : Inport  Port=2
  Iabc : Inport  Port=3
  wt : Inport  Port=4
  Demux : Demux  Outputs=3
  Demux1 : Demux  Outputs=3
  Demux2 : Demux  Outputs=3
  Terminator : Terminator
  Terminator1 : Terminator
  Terminator2 : Terminator
  abc to dq0 : spsabctodq0Lib/abc to dq0  Alignment=90 degrees behind phase A axis
  abc to dq1 : spsabctodq0Lib/abc to dq0  Alignment=90 degrees behind phase A axis
  abc to dq2 : spsabctodq0Lib/abc to dq0  Alignment=90 degrees behind phase A axis
  ILd : Outport
  ILq : Outport  Port=2
  Vd : Outport  Port=3
  Vq : Outport  Port=4
  Id : Outport  Port=5
  Iq : Outport  Port=6
  wires:
  ILabc/1 -> abc to dq0/1
  abc to dq0/1 -> Demux/1
  Demux/3 -> Terminator/1
  Demux/1 -> ILd/1
  Demux/2 -> ILq/1
  Demux1/2 -> Vq/1
  Demux1/1 -> Vd/1
  Demux1/3 -> Terminator1/1
  abc to dq1/1 -> Demux1/1
  Vabc/1 -> abc to dq1/1
  Iabc/1 -> abc to dq2/1
  abc to dq2/1 -> Demux2/1
  Demux2/3 -> Terminator2/1
  Demux2/1 -> Id/1
  Demux2/2 -> Iq/1
  wt/1 -> abc to dq2/2, abc to dq1/2, abc to dq0/2
